simulink model "low_pass_filters"  (R2022b)
settings: Solver=FixedStepAuto  StartTime=0.0  StopTime=50  FixedStep=0.001  RelTol=1e-3
values from neighbouring files (symbols this model uses):
  LP_Filter_Df = 1    [init_LH_filters.m]
  LP_Filter_Tf = 0.001    [init_LH_filters.m]
  LP_FO_Gain_a = 0.5    [init_LH_filters.m]
  LP_FO_Gain_b = 0.5    [init_LH_filters.m]
undefined symbols (not defined in the file or in its folder): DiscIntNeverNeededParam
settings Model: Creator=Z0150218  LastModifiedBy=Z0150218

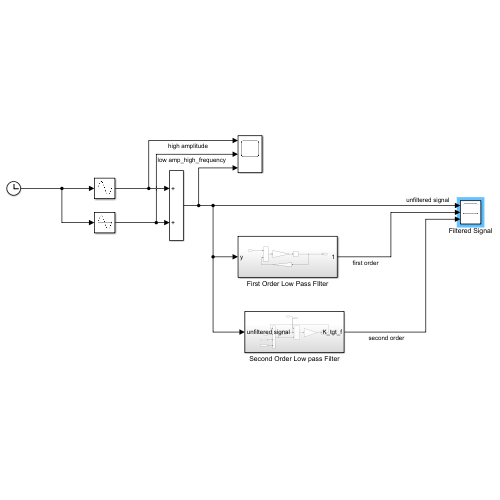
[thumbnail: Simulink's stored preview of the top-level diagram]
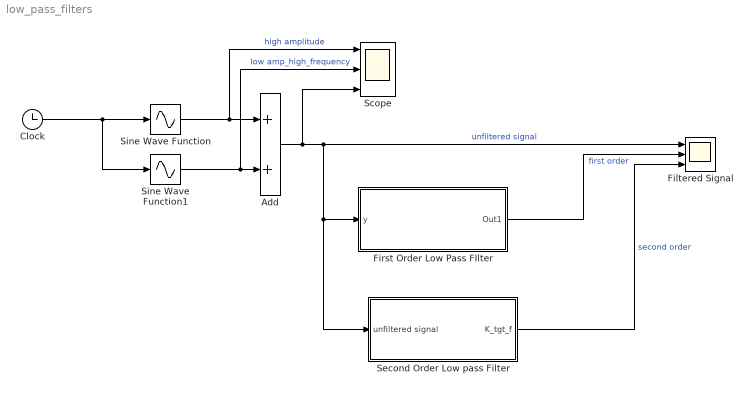
== system low_pass_filters ==
  Add : Sum
  Clock : Clock
  Filtered Signal : Scope  NumInputPorts=3
  First Order Low Pass FIlter : Subsystem
  Scope : Scope  NumInputPorts=3
  Second Order Low pass Filter : Subsystem
  Sine Wave Function : Sin  TimeSource=Use external signal  Amplitude=50  SampleTime=0
  Sine Wave Function1 : Sin  TimeSource=Use external signal  Amplitude=5  Frequency=10  SampleTime=0
  wires:
  Clock/1 -> Sine Wave Function1/1, Sine Wave Function/1
  Add/1 -> Scope/3, Second Order Low pass Filter/1(unfiltered signal), First Order Low Pass FIlter/1(y), Filtered Signal/1  "unfiltered signal"
  Second Order Low pass Filter/1(K_tgt_f) -> Filtered Signal/3  "second order"
  First Order Low Pass FIlter/1(Out1) -> Filtered Signal/2  "first order"
  Sine Wave Function/1 -> Scope/1, Add/1  "high amplitude"
  Sine Wave Function1/1 -> Scope/2, Add/2  "low amp_high_frequency"

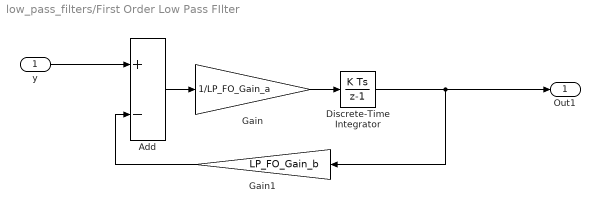
== system low_pass_filters/First Order Low Pass FIlter ==
  y : Inport
  Add : Sum  Inputs=+-
  Discrete-Time Integrator : DiscreteIntegrator  SampleTime=-1  ICPrevOutput=DiscIntNeverNeededParam  ICPrevScaledInput=DiscIntNeverNeededParam
  Gain : Gain  Gain=1/LP_FO_Gain_a
  Gain1 : Gain  Gain=LP_FO_Gain_b
  Out1 : Outport
  wires:
  y/1 -> Add/1
  Discrete-Time Integrator/1 -> Out1/1, Gain1/1
  Add/1 -> Gain/1
  Gain/1 -> Discrete-Time Integrator/1
  Gain1/1 -> Add/2

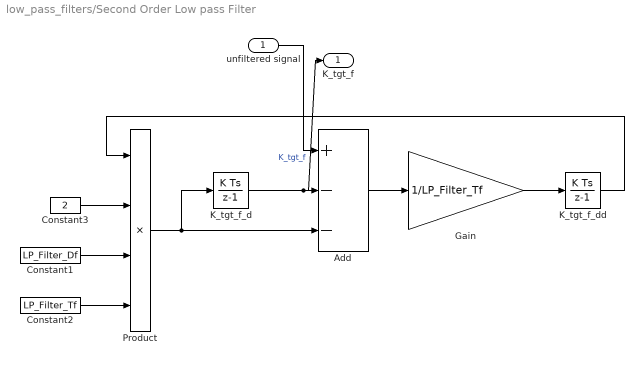
== system low_pass_filters/Second Order Low pass Filter ==
  unfiltered signal : Inport
  Add : Sum  Inputs=+--
  Constant1 : Constant  Value=LP_Filter_Df
  Constant2 : Constant  Value=LP_Filter_Tf
  Constant3 : Constant  Value=2
  Gain : Gain  Gain=1/LP_Filter_Tf
  K_tgt_f_d : DiscreteIntegrator  SampleTime=-1  ICPrevOutput=DiscIntNeverNeededParam  ICPrevScaledInput=DiscIntNeverNeededParam
  K_tgt_f_dd : DiscreteIntegrator  SampleTime=-1  ICPrevOutput=DiscIntNeverNeededParam  ICPrevScaledInput=DiscIntNeverNeededParam
  Product : Product  Inputs=4
  K_tgt_f : Outport
  wires:
  Constant1/1 -> Product/3
  unfiltered signal/1 -> Add/1
  Constant2/1 -> Product/4
  K_tgt_f_dd/1 -> Product/1
  K_tgt_f_d/1 -> K_tgt_f/1, Add/2  "K_tgt_f"
  Product/1 -> Add/3, K_tgt_f_d/1
  Constant3/1 -> Product/2
  Gain/1 -> K_tgt_f_dd/1
  Add/1 -> Gain/1
